simulink model "Motor_Position_Control0"  (R2020b)
settings: Solver=VariableStepAuto  StartTime=0.0  StopTime=120  RelTol=1e-3
undefined symbols (not defined in the file): b, J, K, L, R
settings Model: DataDictionary=Data_Dict_Motor_position.sldd  Creator=intel  LastModifiedBy=intel
settings DataIOCC: SaveOutput=off  SaveTime=off

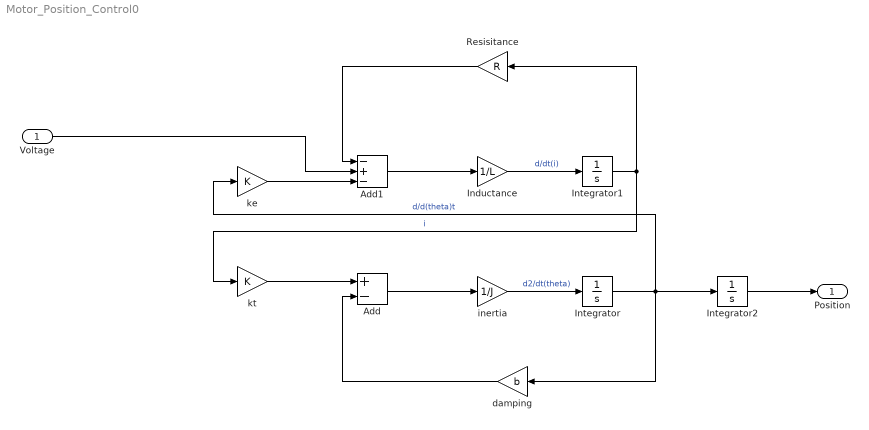
== system Motor_Position_Control0 ==
  Voltage : Inport  OutDataTypeStr=double  PortDimensions=1  SampleTime=0
  " Add" : Sum  Inputs=+-
  " Add1" : Sum  Inputs=-+-
  " Integrator" : Integrator
  " Integrator1" : Integrator
  " Integrator2" : Integrator
  Inductance : Gain  Gain=1/L
  Resisitance : Gain  Gain=R
  damping : Gain  Gain=b
  inertia : Gain  Gain=1/J
  ke : Gain  Gain=K
  kt : Gain  Gain=K
  Position : Outport  OutDataTypeStr=double  PortDimensions=1  SampleTime=0
  wires:
  " Add"/1 -> inertia/1
  " Integrator1"/1 -> kt/1, Resisitance/1  "i"
  Inductance/1 -> " Integrator1"/1  "d/dt(i)"
  ke/1 -> " Add1"/3
  " Integrator2"/1 -> Position/1
  damping/1 -> " Add"/2
  Voltage/1 -> " Add1"/2
  " Integrator"/1 -> damping/1, ke/1, " Integrator2"/1  "d/d(theta)t"
  Resisitance/1 -> " Add1"/1
  " Add1"/1 -> Inductance/1
  kt/1 -> " Add"/1
  inertia/1 -> " Integrator"/1  "d2/dt(theta)"
